simulink model "MPO_braking_system"  (R2021b)
settings: Solver=VariableStepAuto  StartTime=0.0  StopTime=10  FixedStep=0.0001  MaxStep=0.01  RelTol=1e-3  EnableMultiTasking=on
PreLoadFcn:
  | sdl_braking_caliper_disk_brake_input
InitFcn:
  | f10 = 5; f11 = f10; f12 = f10;
  | f20 = 5; f21 = f20; f22 = f20;
undefined symbols (not defined in the file or in its folder): fcdb, tpc
libraries: fl_lib x154, nesl_utility x45, SimscapeFluids_lib x6, sdl_lib x4
(part 1 of 3)
CloseFcn:
  | try,close(h_sdl_braking_caliper_disk_brake),end
  | clear h_sdl_braking_caliper_disk_brake
  | 
  | clear fcdb simT tpc tout
  | clear simlog_sdl_braking_caliper_disk_brake
settings Model: PacingRate=0.100000  Creator=samira  LastModifiedBy=109100
settings SolverCC: AlgebraicLoopSolver=TrustRegion  SolverResetMethod=Robust
settings DataIOCC: LimitDataPoints=on  SaveFormat=Array  ReturnWorkspaceOutputs=off
settings OptimizationCC: LifeSpan=inf
settings DebuggingCC: SolverPrmCheckMsg=warning  SFUnexpectedBacktrackingDiag=warning  SFNoUnconditionalDefaultTransitionDiag=warning  SFExecutionAtInitializationDiag=none  SFMachineParentedDataDiag=warning  ArithmeticOperatorsInVariantConditions=warning
settings HardwareCC: ProdBitPerPointer=32  ProdBitPerSizeT=32  ProdBitPerPtrDiffT=32  ProdLargestAtomicFloat=None  ProdIntDivRoundTo=Undefined  ProdEndianess=Unspecified  ProdWordSize=32  ProdHWDeviceType=32-bit Generic
settings ModelReferenceCC: PropagateSignalLabelsOutOfModel=off
settings SFSimCC: SimUseLocalCustomCode=off  CustomCodeUndefinedFunction=UseInterfaceOnly
settings RTWCC: RTWUseLocalCustomCode=off
settings CodeAppCC: StateflowObjectComments=on
settings GRTTargetCC: TargetLangStandard=C89/C90 (ANSI)
settings ConfigComp: CovMetricSettings=dw  CovSaveCumulativeToWorkspaceVar=on  CovSaveSingleToWorkspaceVar=on  CovExternalEMLEnable=off  CovSFcnEnable=off

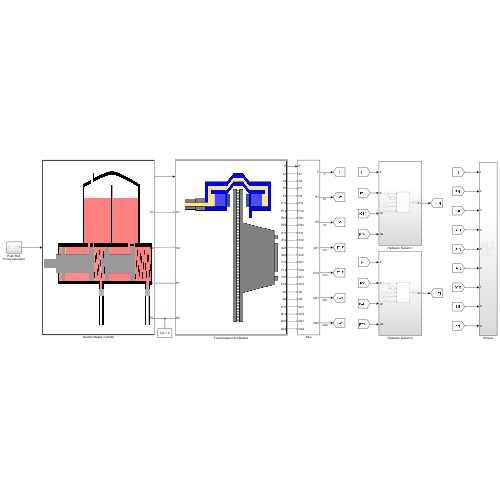
[thumbnail: Simulink's stored preview of the top-level diagram]
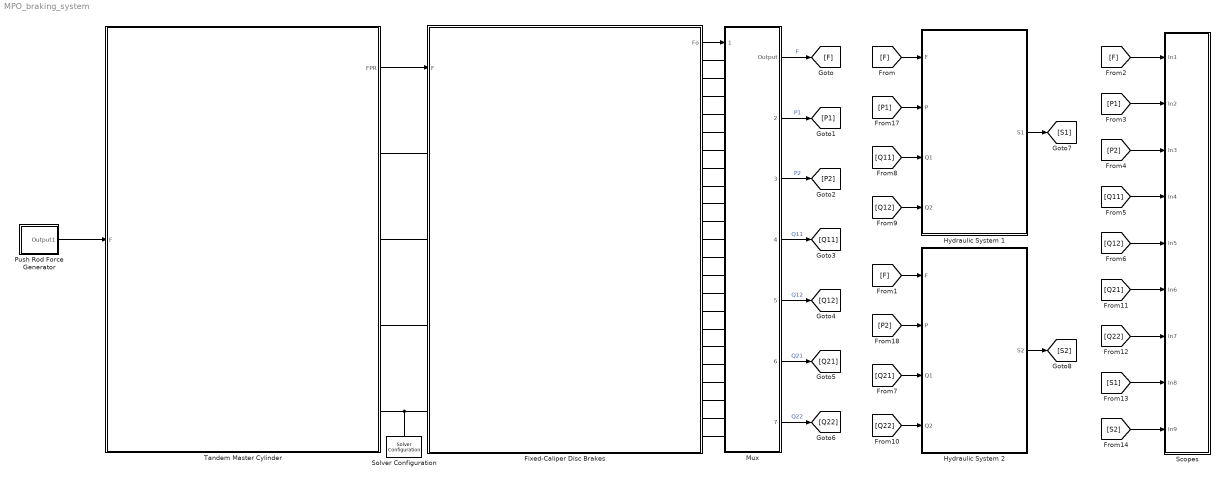
== system MPO_braking_system ==
  Fixed-Caliper Disc Brakes : Subsystem  Tag=ModelFeatures
      mask Display:
      | image('sdl_braking_caliper_disk_brake.png')
      | port_label('output',1,'F')
      | port_label('LConn',1,'X1')
      | port_label('LConn',2,'X2')
      | port_label('LConn',3,'P1')
      | port_label('LConn',4,'P2')
      | port_label('RConn',1,'X1')
      | port_label('RConn',2,'X2')
      | port_label('RConn',3,'P1')
      | port_label('RConn',4,'P2')
      | port_label('RConn',5,'P11')
      | port_label('RConn',6,'P12')
      | port_label('RConn',7,'P21')
      | port_label('RConn',8,'P22')
      | port_label('RConn',9,'X11')
      | port_label('RConn',10,'X12')
      | port_label('RConn',11,'X21')
      | port_label('RConn',12,'X22')
      | port_label('RConn',13,'F11')
      | port_label('RConn',14,'F12')
      | port_label('RConn',15,'F21')
      | port_label('RConn',16,'F22')
      | port_label('RConn',17,'Q1')
      | port_label('RConn',18,'Q2')
      | port_label('RConn',19,'Q11')
      | port_label('RConn',20,'Q12')
      | port_label('RConn',21,'Q21')
      | port_label('RConn',22,'Q22')
  Hydraulic System 1 : Subsystem
  Hydraulic System 2 : Subsystem
  Mux : Subsystem  Tag=ModelFeatures
      mask Display:
      | port_label('input',1,'F')
      | port_label('LConn',1,'S1')
      | port_label('LConn',2,'S2')
      | port_label('LConn',3,'P1')
      | port_label('LConn',4,'P2')
      | port_label('LConn',5,'P11')
      | port_label('LConn',6,'P12')
      | port_label('LConn',7,'P21')
      | port_label('LConn',8,'P22')
      | port_label('LConn',9,'S11')
      | port_label('LConn',10,'S12')
      | port_label('LConn',11,'S11')
      | port_label('LConn',12,'S12')
      | port_label('LConn',13,'Q11')
      | port_label('LConn',14,'Q12')
      | port_label('LConn',15,'Q11')
      | port_label('LConn',16,'Q12')
      | port_label('LConn',17,'Q1')
      | port_label('LConn',18,'Q2')
      | port_label('LConn',19,'Q11')
      | port_label('LConn',20,'Q12')
      | port_label('LConn',21,'Q21')
      | port_label('LConn',22,'Q22')
      | port_label('output',1,'F')
      | port_label('output',2,'P1')
      | port_label('output',3,'P2')
      | port_label('output',4,'Q11')
      | port_label('output',5,'Q12')
      | port_label('output',6,'Q21')
      | port_label('output',7,'Q22')
  Push Rod Force Generator : Subsystem
  Scopes : Subsystem
  Solver Configuration : nesl_utility/Solver Configuration  Tag=ModelFeatures  PhysicalDomain=network_engine_domain  SubClassName=solver  LeftPortType=input  RightPortType=generic  Tones=[]  Harmonics=[]  SimulateNoise=off  Profile=off  UseLocalSampling=off  EnableSwitchedLinearOptims=on  FrequencyDomain=off  UseCCode=off  RelTol=0.001  AbsTol=1e-06  MinStep=1e-09  ToWorkspace=off  RevertToSquareIcSolve=off  NumHomotopyIterations=100  PhasorMode=off  PhasorModeNumHarmonics=1  DoDC=on  ResidualTolerance=1e-09  UseLocalSolver=off  LocalSolverChoice=NE_BACKWARD_EULER_ADVANCER  LocalSolverSampleTime=0.001  DoFixedCost=off  MaxNonlinIter=3  MaxModeIter=2  ComputeImpulses=off  ImpulseIterations=2  LinearAlgebra=auto  EquationFormulation=NE_TIME_EF  DelaysMemoryBudget=1024  AutomaticFiltering=on  FilteringTimeConstant=0.001  PartitionStorageMethod=AS_NEEDED  PartitionMemoryBudget=1024  PartitionMethod=FAST
      settings: SourceProductBaseCode=PW,SS
  Tandem Master Cylinder : Subsystem
      mask Display:
      | image('sdl_braking_tandem_primary_cylinder.png');
      | %port_label('RConn',1,'F')
      | port_label('RConn',1,'X1')
      | port_label('RConn',2,'X2')
      | port_label('RConn',3,'P1')
      | port_label('RConn',4,'P2')
  wires:
  Push Rod Force Generator/1(Output1) -> Tandem Master Cylinder/1(F)
  Mux/4(Output3) -> [Q11]  "Q11"
  Tandem Master Cylinder/1(FPR) -> Fixed-Caliper Disc Brakes/1(F)
  Fixed-Caliper Disc Brakes/1(Fo) -> Mux/1(input01)
  Mux/1(Output) -> [F]  "F"
  Mux/5(Output4) -> [Q12]  "Q12"
  Mux/7(Output6) -> [Q22]  "Q22"
  Mux/6(Output5) -> [Q21]  "Q21"
  [F] -> Hydraulic System 1/1(F)
  [Q12] -> Hydraulic System 1/4(Q2)
  [Q21] -> Hydraulic System 2/3(Q1)
  [F] -> Hydraulic System 2/1(F)
  [Q22] -> Hydraulic System 2/4(Q2)
  Mux/2(Output1) -> [P1]  "P1"
  Mux/3(Output2) -> [P2]  "P2"
  [P1] -> Hydraulic System 1/2(P)
  [Q11] -> Hydraulic System 1/3(Q1)
  [P2] -> Hydraulic System 2/2(P)
  Hydraulic System 1/1(S1) -> [S1]
  Hydraulic System 2/1(S2) -> [S2]
  [F] -> Scopes/1(In1)
  [P1] -> Scopes/2(In2)
  [P2] -> Scopes/3(In3)
  [Q11] -> Scopes/4(In4)
  [Q12] -> Scopes/5(In5)
  [Q21] -> Scopes/6(In6)
  [Q22] -> Scopes/7(In7)
  [S1] -> Scopes/8(In8)
  [S2] -> Scopes/9(In9)
  connections:
  Fixed-Caliper Disc Brakes/LConn4 -- Tandem Master Cylinder/RConn4 -- Solver Configuration/RConn1
  Mux/LConn3 -- Fixed-Caliper Disc Brakes/RConn3
  Fixed-Caliper Disc Brakes/RConn19 -- Mux/LConn19
  Fixed-Caliper Disc Brakes/RConn20 -- Mux/LConn20
  Fixed-Caliper Disc Brakes/RConn21 -- Mux/LConn21
  Fixed-Caliper Disc Brakes/LConn3 -- Tandem Master Cylinder/RConn3
  Tandem Master Cylinder/RConn1 -- Fixed-Caliper Disc Brakes/LConn1
  Mux/LConn4 -- Fixed-Caliper Disc Brakes/RConn4
  Tandem Master Cylinder/RConn2 -- Fixed-Caliper Disc Brakes/LConn2
  Fixed-Caliper Disc Brakes/RConn18 -- Mux/LConn18
  Fixed-Caliper Disc Brakes/RConn17 -- Mux/LConn17
  Fixed-Caliper Disc Brakes/RConn16 -- Mux/LConn16
  Fixed-Caliper Disc Brakes/RConn15 -- Mux/LConn15
  Fixed-Caliper Disc Brakes/RConn14 -- Mux/LConn14
  Fixed-Caliper Disc Brakes/RConn13 -- Mux/LConn13
  Mux/LConn12 -- Fixed-Caliper Disc Brakes/RConn12
  Fixed-Caliper Disc Brakes/RConn11 -- Mux/LConn11
  Fixed-Caliper Disc Brakes/RConn10 -- Mux/LConn10
  Fixed-Caliper Disc Brakes/RConn9 -- Mux/LConn9
  Fixed-Caliper Disc Brakes/RConn1 -- Mux/LConn1
  Fixed-Caliper Disc Brakes/RConn2 -- Mux/LConn2
  Fixed-Caliper Disc Brakes/RConn5 -- Mux/LConn5
  Fixed-Caliper Disc Brakes/RConn6 -- Mux/LConn6
  Fixed-Caliper Disc Brakes/RConn7 -- Mux/LConn7
  Fixed-Caliper Disc Brakes/RConn8 -- Mux/LConn8
  Fixed-Caliper Disc Brakes/RConn22 -- Mux/LConn22

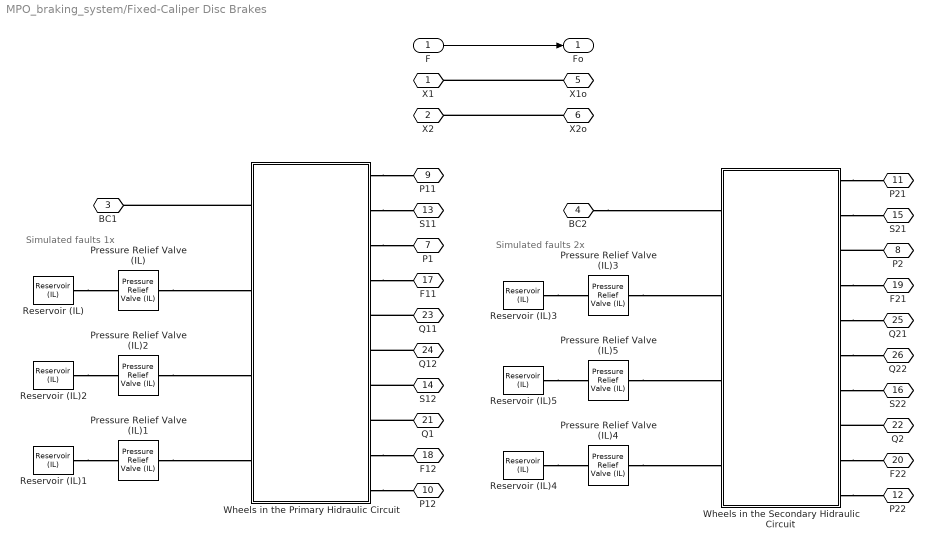
== system MPO_braking_system/Fixed-Caliper Disc Brakes ==
  note: Simulated faults 1x
  note: Simulated faults 2x
  F : Inport
  Pressure Relief Valve (IL) : SimscapeFluids_lib/Isothermal Liquid/Valves & Orifices/Pressure Control Valves/Pressure Relief Valve (IL)  set_pressure_spec=foundation.enum.constant_controlled.constant  pressure_spec=fluids.isothermal_liquid.valves_orifices.enum.pressure_control_spec.dp  p_set_gauge=0.1 MPa  p_set_differential=f10 MPa  p_range=0.1 MPa  opening_spec=fluids.isothermal_liquid.valves_orifices.enum.opening_spec.linear  area_max=1e-4 m^2  area_leak=1e-10 m^2  p_diff_TLU=[0.2 : 0.2 : 1.2] MPa  valve_area_TLU=[1e-10, 2e-06, 4e-06, 6e-06, 8e-06, 1e-05] m^2  area=inf m^2  Cd=0.64  Re_c=150  pressure_recovery=simscape.enum.onoff.off  smoothing_factor=0.01  opening_dynamics=simscape.enum.onoff.off  tau=0.1 s  enable_faults=simscape.enum.onoff.off  fault_type=fluids.enum.FaultOpening.Closed  fault_trigger=foundation.enum.faultSpec.Temporal  fault_time=5 s
      settings: SourceProductBaseCode=SH  InternalSimscapePortConfiguration="{\"Bottom\":[],\"Left\":[{\"id\":\"A\",\"label\":\"A\",\"type\":\"foundation.isothermal_liquid.isothermal_liquid\"}],\"Right\":[{\"id\":\"B\",\"label\":\"B\",\"type\":\"foundation.isothermal_liquid.isothermal_liquid\"}],\"Top\":[]}"
  Pressure Relief Valve (IL)1 : SimscapeFluids_lib/Isothermal Liquid/Valves & Orifices/Pressure Control Valves/Pressure Relief Valve (IL)  set_pressure_spec=foundation.enum.constant_controlled.constant  pressure_spec=fluids.isothermal_liquid.valves_orifices.enum.pressure_control_spec.dp  p_set_gauge=0.1 MPa  p_set_differential=f12 MPa  p_range=0.1 MPa  opening_spec=fluids.isothermal_liquid.valves_orifices.enum.opening_spec.linear  area_max=1e-4 m^2  area_leak=1e-10 m^2  p_diff_TLU=[0.2 : 0.2 : 1.2] MPa  valve_area_TLU=[1e-10, 2e-06, 4e-06, 6e-06, 8e-06, 1e-05] m^2  area=inf m^2  Cd=0.64  Re_c=150  pressure_recovery=simscape.enum.onoff.off  smoothing_factor=0.01  opening_dynamics=simscape.enum.onoff.off  tau=0.1 s  enable_faults=simscape.enum.onoff.off  fault_type=fluids.enum.FaultOpening.Closed  fault_trigger=foundation.enum.faultSpec.Temporal  fault_time=5 s
      settings: SourceProductBaseCode=SH  InternalSimscapePortConfiguration="{\"Bottom\":[],\"Left\":[{\"id\":\"A\",\"label\":\"A\",\"type\":\"foundation.isothermal_liquid.isothermal_liquid\"}],\"Right\":[{\"id\":\"B\",\"label\":\"B\",\"type\":\"foundation.isothermal_liquid.isothermal_liquid\"}],\"Top\":[]}"
  Pressure Relief Valve (IL)2 : SimscapeFluids_lib/Isothermal Liquid/Valves & Orifices/Pressure Control Valves/Pressure Relief Valve (IL)  set_pressure_spec=foundation.enum.constant_controlled.constant  pressure_spec=fluids.isothermal_liquid.valves_orifices.enum.pressure_control_spec.dp  p_set_gauge=0.1 MPa  p_set_differential=f11 MPa  p_range=0.1 MPa  opening_spec=fluids.isothermal_liquid.valves_orifices.enum.opening_spec.linear  area_max=1e-4 m^2  area_leak=1e-10 m^2  p_diff_TLU=[0.2 : 0.2 : 1.2] MPa  valve_area_TLU=[1e-10, 2e-06, 4e-06, 6e-06, 8e-06, 1e-05] m^2  area=inf m^2  Cd=0.64  Re_c=150  pressure_recovery=simscape.enum.onoff.off  smoothing_factor=0.01  opening_dynamics=simscape.enum.onoff.off  tau=0.1 s  enable_faults=simscape.enum.onoff.off  fault_type=fluids.enum.FaultOpening.Closed  fault_trigger=foundation.enum.faultSpec.Temporal  fault_time=5 s
      settings: SourceProductBaseCode=SH  InternalSimscapePortConfiguration="{\"Bottom\":[],\"Left\":[{\"id\":\"A\",\"label\":\"A\",\"type\":\"foundation.isothermal_liquid.isothermal_liquid\"}],\"Right\":[{\"id\":\"B\",\"label\":\"B\",\"type\":\"foundation.isothermal_liquid.isothermal_liquid\"}],\"Top\":[]}"
  Pressure Relief Valve (IL)3 : SimscapeFluids_lib/Isothermal Liquid/Valves & Orifices/Pressure Control Valves/Pressure Relief Valve (IL)  set_pressure_spec=foundation.enum.constant_controlled.constant  pressure_spec=fluids.isothermal_liquid.valves_orifices.enum.pressure_control_spec.dp  p_set_gauge=0.1 MPa  p_set_differential=f20 MPa  p_range=0.1 MPa  opening_spec=fluids.isothermal_liquid.valves_orifices.enum.opening_spec.linear  area_max=1e-4 m^2  area_leak=1e-10 m^2  p_diff_TLU=[0.2 : 0.2 : 1.2] MPa  valve_area_TLU=[1e-10, 2e-06, 4e-06, 6e-06, 8e-06, 1e-05] m^2  area=inf m^2  Cd=0.64  Re_c=150  pressure_recovery=simscape.enum.onoff.off  smoothing_factor=0.01  opening_dynamics=simscape.enum.onoff.off  tau=0.1 s  enable_faults=simscape.enum.onoff.off  fault_type=fluids.enum.FaultOpening.Closed  fault_trigger=foundation.enum.faultSpec.Temporal  fault_time=5 s
      settings: SourceProductBaseCode=SH  InternalSimscapePortConfiguration="{\"Bottom\":[],\"Left\":[{\"id\":\"A\",\"label\":\"A\",\"type\":\"foundation.isothermal_liquid.isothermal_liquid\"}],\"Right\":[{\"id\":\"B\",\"label\":\"B\",\"type\":\"foundation.isothermal_liquid.isothermal_liquid\"}],\"Top\":[]}"
  Pressure Relief Valve (IL)4 : SimscapeFluids_lib/Isothermal Liquid/Valves & Orifices/Pressure Control Valves/Pressure Relief Valve (IL)  set_pressure_spec=foundation.enum.constant_controlled.constant  pressure_spec=fluids.isothermal_liquid.valves_orifices.enum.pressure_control_spec.dp  p_set_gauge=0.1 MPa  p_set_differential=f22 MPa  p_range=0.1 MPa  opening_spec=fluids.isothermal_liquid.valves_orifices.enum.opening_spec.linear  area_max=1e-4 m^2  area_leak=1e-10 m^2  p_diff_TLU=[0.2 : 0.2 : 1.2] MPa  valve_area_TLU=[1e-10, 2e-06, 4e-06, 6e-06, 8e-06, 1e-05] m^2  area=inf m^2  Cd=0.64  Re_c=150  pressure_recovery=simscape.enum.onoff.off  smoothing_factor=0.01  opening_dynamics=simscape.enum.onoff.off  tau=0.1 s  enable_faults=simscape.enum.onoff.off  fault_type=fluids.enum.FaultOpening.Closed  fault_trigger=foundation.enum.faultSpec.Temporal  fault_time=5 s
      settings: SourceProductBaseCode=SH  InternalSimscapePortConfiguration="{\"Bottom\":[],\"Left\":[{\"id\":\"A\",\"label\":\"A\",\"type\":\"foundation.isothermal_liquid.isothermal_liquid\"}],\"Right\":[{\"id\":\"B\",\"label\":\"B\",\"type\":\"foundation.isothermal_liquid.isothermal_liquid\"}],\"Top\":[]}"
  Pressure Relief Valve (IL)5 : SimscapeFluids_lib/Isothermal Liquid/Valves & Orifices/Pressure Control Valves/Pressure Relief Valve (IL)  set_pressure_spec=foundation.enum.constant_controlled.constant  pressure_spec=fluids.isothermal_liquid.valves_orifices.enum.pressure_control_spec.dp  p_set_gauge=0.1 MPa  p_set_differential=f21 MPa  p_range=0.1 MPa  opening_spec=fluids.isothermal_liquid.valves_orifices.enum.opening_spec.linear  area_max=1e-4 m^2  area_leak=1e-10 m^2  p_diff_TLU=[0.2 : 0.2 : 1.2] MPa  valve_area_TLU=[1e-10, 2e-06, 4e-06, 6e-06, 8e-06, 1e-05] m^2  area=inf m^2  Cd=0.64  Re_c=150  pressure_recovery=simscape.enum.onoff.off  smoothing_factor=0.01  opening_dynamics=simscape.enum.onoff.off  tau=0.1 s  enable_faults=simscape.enum.onoff.off  fault_type=fluids.enum.FaultOpening.Closed  fault_trigger=foundation.enum.faultSpec.Temporal  fault_time=5 s
      settings: SourceProductBaseCode=SH  InternalSimscapePortConfiguration="{\"Bottom\":[],\"Left\":[{\"id\":\"A\",\"label\":\"A\",\"type\":\"foundation.isothermal_liquid.isothermal_liquid\"}],\"Right\":[{\"id\":\"B\",\"label\":\"B\",\"type\":\"foundation.isothermal_liquid.isothermal_liquid\"}],\"Top\":[]}"
  Reservoir (IL){,1..5} (6 alike) : fl_lib/Isothermal Liquid/Elements/Reservoir (IL)  reservoir_type=foundation.enum.constant_controlled.constant  pressure_spec=foundation.enum.pressure_spec.atmospheric  reservoir_pressure=0.101325 MPa
      settings: SourceProductBaseCode=SS
  Wheels in the Primary Hidraulic Circuit : Subsystem
  Wheels in the Secondary Hidraulic Circuit : Subsystem
  X1 : PMIOPort  Side=Left
  X2 : PMIOPort  Port=2  Side=Left
  BC1 : PMIOPort  Port=3  Side=Left
  BC2 : PMIOPort  Port=4  Side=Left
  X1o : PMIOPort  Port=5  Side=Right
  X2o : PMIOPort  Port=6  Side=Right
  P1 : PMIOPort  Port=7  Side=Right
  P2 : PMIOPort  Port=8  Side=Right
  P11 : PMIOPort  Port=9  Side=Right
  P12 : PMIOPort  Port=10  Side=Right
  P21 : PMIOPort  Port=11  Side=Right
  P22 : PMIOPort  Port=12  Side=Right
  S11 : PMIOPort  Port=13  Side=Right
  S12 : PMIOPort  Port=14  Side=Right
  S21 : PMIOPort  Port=15  Side=Right
  S22 : PMIOPort  Port=16  Side=Right
  F11 : PMIOPort  Port=17  Side=Right
  F12 : PMIOPort  Port=18  Side=Right
  F21 : PMIOPort  Port=19  Side=Right
  F22 : PMIOPort  Port=20  Side=Right
  Q1 : PMIOPort  Port=21  Side=Right
  Q2 : PMIOPort  Port=22  Side=Right
  Q11 : PMIOPort  Port=23  Side=Right
  Q12 : PMIOPort  Port=24  Side=Right
  Q21 : PMIOPort  Port=25  Side=Right
  Q22 : PMIOPort  Port=26  Side=Right
  Fo : Outport
  wires:
  F/1 -> Fo/1
  connections:
  X1o/RConn1 -- X1/RConn1
  X2o/RConn1 -- X2/RConn1
  Reservoir (IL)/LConn1 -- Pressure Relief Valve (IL)/RConn1
  Reservoir (IL)2/LConn1 -- Pressure Relief Valve (IL)2/RConn1
  Reservoir (IL)1/LConn1 -- Pressure Relief Valve (IL)1/RConn1
  Reservoir (IL)5/LConn1 -- Pressure Relief Valve (IL)5/RConn1
  Reservoir (IL)3/LConn1 -- Pressure Relief Valve (IL)3/RConn1
  Reservoir (IL)4/LConn1 -- Pressure Relief Valve (IL)4/RConn1
  Wheels in the Primary Hidraulic Circuit/RConn1 -- P11/RConn1
  Wheels in the Primary Hidraulic Circuit/RConn2 -- S11/RConn1
  Wheels in the Primary Hidraulic Circuit/RConn3 -- P1/RConn1
  Wheels in the Primary Hidraulic Circuit/RConn4 -- F11/RConn1
  Q11/RConn1 -- Wheels in the Primary Hidraulic Circuit/RConn5
  Wheels in the Primary Hidraulic Circuit/LConn1 -- BC1/RConn1
  Q12/RConn1 -- Wheels in the Primary Hidraulic Circuit/RConn6
  S12/RConn1 -- Wheels in the Primary Hidraulic Circuit/RConn7
  Q1/RConn1 -- Wheels in the Primary Hidraulic Circuit/RConn8
  Wheels in the Primary Hidraulic Circuit/RConn9 -- F12/RConn1
  Wheels in the Primary Hidraulic Circuit/RConn10 -- P12/RConn1
  Pressure Relief Valve (IL)/LConn1 -- Wheels in the Primary Hidraulic Circuit/LConn2
  Pressure Relief Valve (IL)2/LConn1 -- Wheels in the Primary Hidraulic Circuit/LConn3
  Pressure Relief Valve (IL)1/LConn1 -- Wheels in the Primary Hidraulic Circuit/LConn4
  Wheels in the Secondary Hidraulic Circuit/RConn1 -- P21/RConn1
  Wheels in the Secondary Hidraulic Circuit/RConn2 -- S21/RConn1
  P2/RConn1 -- Wheels in the Secondary Hidraulic Circuit/RConn3
  Wheels in the Secondary Hidraulic Circuit/RConn4 -- F21/RConn1
  Wheels in the Secondary Hidraulic Circuit/RConn5 -- Q21/RConn1
  BC2/RConn1 -- Wheels in the Secondary Hidraulic Circuit/LConn1
  Wheels in the Secondary Hidraulic Circuit/RConn6 -- Q22/RConn1
  Wheels in the Secondary Hidraulic Circuit/RConn7 -- S22/RConn1
  Q2/RConn1 -- Wheels in the Secondary Hidraulic Circuit/RConn8
  Wheels in the Secondary Hidraulic Circuit/RConn9 -- F22/RConn1
  Wheels in the Secondary Hidraulic Circuit/RConn10 -- P22/RConn1
  Pressure Relief Valve (IL)3/LConn1 -- Wheels in the Secondary Hidraulic Circuit/LConn2
  Pressure Relief Valve (IL)5/LConn1 -- Wheels in the Secondary Hidraulic Circuit/LConn3
  Pressure Relief Valve (IL)4/LConn1 -- Wheels in the Secondary Hidraulic Circuit/LConn4

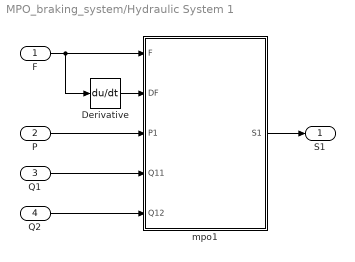
== system MPO_braking_system/Hydraulic System 1 ==
  F : Inport
  P : Inport  Port=2
  Q1 : Inport  Port=3
  Q2 : Inport  Port=4
  Derivative : Derivative
  mpo1 : Stateflow chart  TreatAsAtomicUnit=on
  S1 : Outport
  wires:
  Derivative/1 -> mpo1/2(DF)
  Q2/1 -> mpo1/5(Q12)
  F/1 -> mpo1/1(F), Derivative/1
  Q1/1 -> mpo1/4(Q11)
  P/1 -> mpo1/3(P1)
  mpo1/1(S1) -> S1/1

== system MPO_braking_system/Hydraulic System 2 ==
  F : Inport
  P : Inport  Port=2
  Q1 : Inport  Port=3
  Q2 : Inport  Port=4
  Derivative : Derivative
  mpo2 : Stateflow chart  TreatAsAtomicUnit=on
  S2 : Outport
  wires:
  Derivative/1 -> mpo2/2(DF)
  Q2/1 -> mpo2/5(Q12)
  F/1 -> mpo2/1(F), Derivative/1
  Q1/1 -> mpo2/4(Q11)
  P/1 -> mpo2/3(P1)
  mpo2/1(S2) -> S2/1

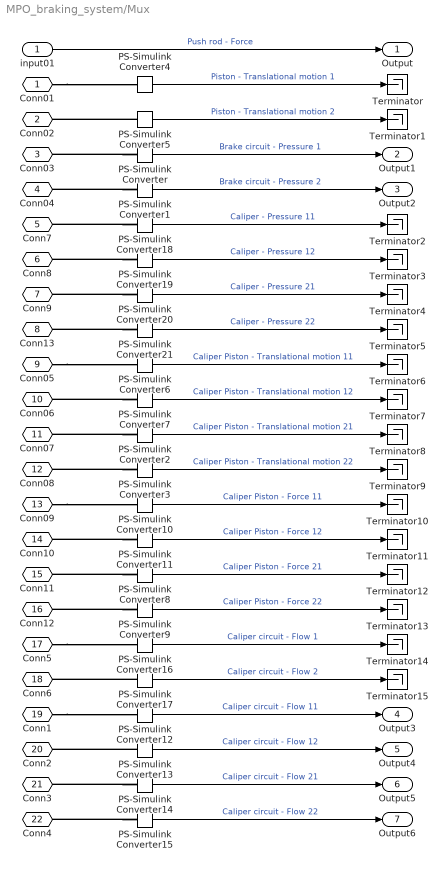
== system MPO_braking_system/Mux ==
  input01 : Inport
  PS-Simulink Converter{,1,18..21} (6 alike) : nesl_utility/PS-Simulink Converter  PhysicalDomain=network_engine_domain  SubClassName=ps_output  LeftPortType=input  RightPortType=output  PseudoPeriodic=off  Frequencies=[]  Unit=Pa  AffineConversion=off
      settings: SourceProductBaseCode=PW,SS
  PS-Simulink Converter{8..11} (4 alike) : nesl_utility/PS-Simulink Converter  PhysicalDomain=network_engine_domain  SubClassName=ps_output  LeftPortType=input  RightPortType=output  PseudoPeriodic=off  Frequencies=[]  Unit=N  AffineConversion=off
      settings: SourceProductBaseCode=PW,SS
  PS-Simulink Converter{12..17} (6 alike) : nesl_utility/PS-Simulink Converter  PhysicalDomain=network_engine_domain  SubClassName=ps_output  LeftPortType=input  RightPortType=output  PseudoPeriodic=off  Frequencies=[]  Unit=m^3/s  AffineConversion=off
      settings: SourceProductBaseCode=PW,SS
  PS-Simulink Converter{2..7} (6 alike) : nesl_utility/PS-Simulink Converter  PhysicalDomain=network_engine_domain  SubClassName=ps_output  LeftPortType=input  RightPortType=output  PseudoPeriodic=off  Frequencies=[]  Unit=m  AffineConversion=off
      settings: SourceProductBaseCode=PW,SS
  Terminator{,1..15} (16 alike) : Terminator
  Conn01 : PMIOPort  Side=Left
  Conn02 : PMIOPort  Port=2  Side=Left
  Conn03 : PMIOPort  Port=3  Side=Left
  Conn04 : PMIOPort  Port=4  Side=Left
  Conn7 : PMIOPort  Port=5  Side=Left
  Conn8 : PMIOPort  Port=6  Side=Left
  Conn9 : PMIOPort  Port=7  Side=Left
  Conn13 : PMIOPort  Port=8  Side=Left
  Conn05 : PMIOPort  Port=9  Side=Left
  Conn06 : PMIOPort  Port=10  Side=Left
  Conn07 : PMIOPort  Port=11  Side=Left
  Conn08 : PMIOPort  Port=12  Side=Left
  Conn09 : PMIOPort  Port=13  Side=Left
  Conn10 : PMIOPort  Port=14  Side=Left
  Conn11 : PMIOPort  Port=15  Side=Left
  Conn12 : PMIOPort  Port=16  Side=Left
  Conn5 : PMIOPort  Port=17  Side=Left
  Conn6 : PMIOPort  Port=18  Side=Left
  Conn1 : PMIOPort  Port=19  Side=Left
  Conn2 : PMIOPort  Port=20  Side=Left
  Conn3 : PMIOPort  Port=21  Side=Left
  Conn4 : PMIOPort  Port=22  Side=Left
  Output : Outport
  Output1 : Outport  Port=2
  Output2 : Outport  Port=3
  Output3 : Outport  Port=4
  Output4 : Outport  Port=5
  Output5 : Outport  Port=6
  Output6 : Outport  Port=7
  wires:
  PS-Simulink Converter/1 -> Output1/1  "Brake circuit - Pressure 1"
  PS-Simulink Converter4/1 -> Terminator/1  "Piston - Translational motion 1"
  input01/1 -> Output/1  "Push rod - Force"
  PS-Simulink Converter10/1 -> Terminator10/1  "Caliper Piston - Force 11"
  PS-Simulink Converter1/1 -> Output2/1  "Brake circuit - Pressure 2"
  PS-Simulink Converter11/1 -> Terminator11/1  "Caliper Piston - Force 12"
  PS-Simulink Converter8/1 -> Terminator12/1  "Caliper Piston - Force 21"
  PS-Simulink Converter9/1 -> Terminator13/1  "Caliper Piston - Force 22"
  PS-Simulink Converter6/1 -> Terminator6/1  "Caliper Piston - Translational motion 11"
  PS-Simulink Converter7/1 -> Terminator7/1  "Caliper Piston - Translational motion 12"
  PS-Simulink Converter2/1 -> Terminator8/1  "Caliper Piston - Translational motion 21"
  PS-Simulink Converter3/1 -> Terminator9/1  "Caliper Piston - Translational motion 22"
  PS-Simulink Converter12/1 -> Output3/1  "Caliper circuit - Flow 11"
  PS-Simulink Converter13/1 -> Output4/1  "Caliper circuit - Flow 12"
  PS-Simulink Converter14/1 -> Output5/1  "Caliper circuit - Flow 21"
  PS-Simulink Converter15/1 -> Output6/1  "Caliper circuit - Flow 22"
  PS-Simulink Converter16/1 -> Terminator14/1  "Caliper circuit - Flow 1"
  PS-Simulink Converter17/1 -> Terminator15/1  "Caliper circuit - Flow 2"
  PS-Simulink Converter19/1 -> Terminator3/1  "Caliper - Pressure 12"
  PS-Simulink Converter18/1 -> Terminator2/1  "Caliper - Pressure 11"
  PS-Simulink Converter21/1 -> Terminator5/1  "Caliper - Pressure 22"
  PS-Simulink Converter20/1 -> Terminator4/1  "Caliper - Pressure 21"
  PS-Simulink Converter5/1 -> Terminator1/1  "Piston - Translational motion 2"
  connections:
  PS-Simulink Converter/LConn1 -- Conn03/RConn1
  PS-Simulink Converter1/LConn1 -- Conn04/RConn1
  PS-Simulink Converter5/LConn1 -- Conn02/RConn1
  Conn01/RConn1 -- PS-Simulink Converter4/LConn1
  PS-Simulink Converter7/LConn1 -- Conn06/RConn1
  PS-Simulink Converter2/LConn1 -- Conn07/RConn1
  Conn05/RConn1 -- PS-Simulink Converter6/LConn1
  PS-Simulink Converter3/LConn1 -- Conn08/RConn1
  PS-Simulink Converter11/LConn1 -- Conn10/RConn1
  PS-Simulink Converter8/LConn1 -- Conn11/RConn1
  PS-Simulink Converter9/LConn1 -- Conn12/RConn1
  Conn09/RConn1 -- PS-Simulink Converter10/LConn1
  PS-Simulink Converter14/LConn1 -- Conn3/RConn1
  Conn1/RConn1 -- PS-Simulink Converter12/LConn1
  PS-Simulink Converter13/LConn1 -- Conn2/RConn1
  PS-Simulink Converter15/LConn1 -- Conn4/RConn1
  PS-Simulink Converter17/LConn1 -- Conn6/RConn1
  Conn5/RConn1 -- PS-Simulink Converter16/LConn1
  PS-Simulink Converter19/LConn1 -- Conn8/RConn1
  PS-Simulink Converter18/LConn1 -- Conn7/RConn1
  PS-Simulink Converter21/LConn1 -- Conn13/RConn1
  PS-Simulink Converter20/LConn1 -- Conn9/RConn1

== system MPO_braking_system/Push Rod Force Generator ==
  Clock : Clock
  Constant : Constant  Value=10e3
  Force Generation : MATLAB Function  TreatAsAtomicUnit=on
  Saturation : Saturate  UpperLimit=tpc.pushRodF(3)  LowerLimit=0
  Stop Simulation : Stop
  Output1 : Outport
  wires:
  Saturation/1 -> Output1/1
  Clock/1 -> Force Generation/1(clock)
  Force Generation/2(signal) -> Saturation/1
  Force Generation/1(stop) -> Stop Simulation/1
  Constant/1 -> Force Generation/2(rate)

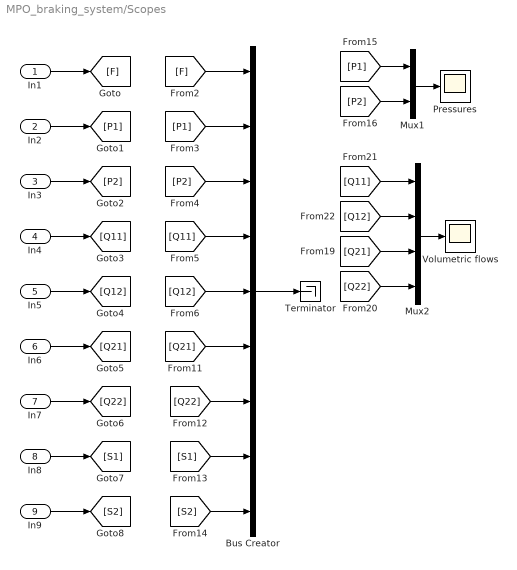
== system MPO_braking_system/Scopes ==
  In1 : Inport
  In2 : Inport  Port=2
  In3 : Inport  Port=3
  In4 : Inport  Port=4
  In5 : Inport  Port=5
  In6 : Inport  Port=6
  In7 : Inport  Port=7
  In8 : Inport  Port=8
  In9 : Inport  Port=9
  Bus Creator : BusCreator  Inputs=9
  Mux1 : Mux  Inputs=2
  Mux2 : Mux
  Pressures : Scope
  Terminator : Terminator
  Volumetric flows : Scope
  wires:
  [Q12] -> Mux2/2
  Bus Creator/1 -> Terminator/1
  In3/1 -> [P2]
  [Q21] -> Mux2/3
  Mux2/1 -> Volumetric flows/1
  In6/1 -> [Q21]
  [Q22] -> Mux2/4
  [P2] -> Mux1/2
  [Q11] -> Mux2/1
  [P1] -> Mux1/1
  In8/1 -> [S1]
  Mux1/1 -> Pressures/1
  In2/1 -> [P1]
  In4/1 -> [Q11]
  In1/1 -> [F]
  In5/1 -> [Q12]
  [S1] -> Bus Creator/8
  [Q21] -> Bus Creator/6
  [Q11] -> Bus Creator/4
  [Q12] -> Bus Creator/5
  [F] -> Bus Creator/1
  [P2] -> Bus Creator/3
  [Q22] -> Bus Creator/7
  [P1] -> Bus Creator/2
  [S2] -> Bus Creator/9
  In7/1 -> [Q22]
  In9/1 -> [S2]

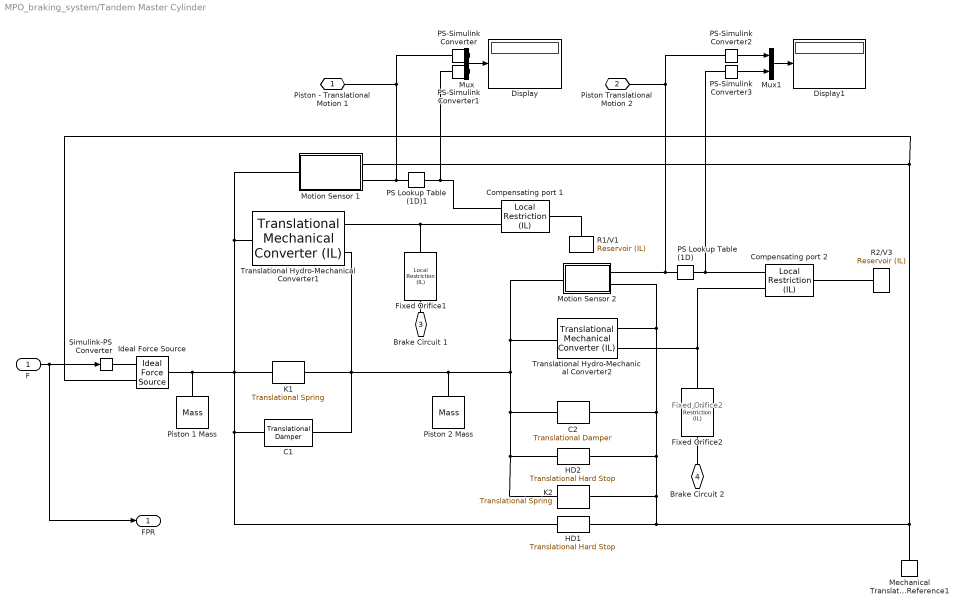
== system MPO_braking_system/Tandem Master Cylinder ==
  note: Fixed Orifice2
  F : Inport
  C1 : fl_lib/Mechanical/Translational Elements/Translational Damper  D=tpc.c1 N/(m/s)  v_specify=off  v_priority=None  v=0 m/s  v_nominal_specify=off  v_nominal_unit=m/s  v_nominal_value=1  f_specify=off  f_priority=None  f=0 N  f_nominal_specify=off  f_nominal_unit=N  f_nominal_value=1
  C2 : fl_lib/Mechanical/Translational Elements/Translational Damper  D=tpc.c2 N/(m/s)  v_specify=off  v_priority=None  v=0 m/s  v_nominal_specify=off  v_nominal_unit=m/s  v_nominal_value=1  f_specify=off  f_priority=None  f=0 N  f_nominal_specify=off  f_nominal_unit=N  f_nominal_value=1
  Compensating port 1 : fl_lib/Isothermal Liquid/Elements/Local Restriction (IL)  restriction_type=foundation.enum.restriction_type.variable  restriction_area=1e-3 m^2  min_area=1e-15 m^2  max_area="tpc.a1Ori  m^2"  area=inf m^2  Cd=0.7  Re_c=150  pressure_recovery=simscape.enum.onoff.off
      settings: SourceProductBaseCode=SS  InternalSimscapePortConfiguration="{\"Bottom\":[],\"Left\":[{\"id\":\"A\",\"label\":\"A\",\"type\":\"foundation.isothermal_liquid.isothermal_liquid\"},{\"id\":\"AR\",\"label\":\"AR\",\"type\":\"input\"}],\"Right\":[{\"id\":\"B\",\"label\":\"B\",\"type\":\"foundation.isothermal_liquid.isothermal_liquid\"}],\"Top\":[]}"
  Compensating port 2 : fl_lib/Isothermal Liquid/Elements/Local Restriction (IL)  restriction_type=foundation.enum.restriction_type.variable  restriction_area=1e-3 m^2  min_area=1e-15 m^2  max_area="tpc.a1Ori  m^2"  area=inf m^2  Cd=0.7  Re_c=150  pressure_recovery=simscape.enum.onoff.off
      settings: SourceProductBaseCode=SS  InternalSimscapePortConfiguration="{\"Bottom\":[],\"Left\":[{\"id\":\"A\",\"label\":\"A\",\"type\":\"foundation.isothermal_liquid.isothermal_liquid\"},{\"id\":\"AR\",\"label\":\"AR\",\"type\":\"input\"}],\"Right\":[{\"id\":\"B\",\"label\":\"B\",\"type\":\"foundation.isothermal_liquid.isothermal_liquid\"}],\"Top\":[]}"
  Display : Display
  Display1 : Display
  Fixed Orifice1 : fl_lib/Isothermal Liquid/Elements/Local Restriction (IL)  restriction_type=foundation.enum.restriction_type.fixed  restriction_area=tpc.a2Ori m^2  min_area=1e-15 m^2  max_area="tpc.a1Ori  m^2"  area=inf m^2  Cd=0.7  Re_c=150  pressure_recovery=simscape.enum.onoff.off
      settings: SourceProductBaseCode=SS  InternalSimscapePortConfiguration="{\"Bottom\":[],\"Left\":[{\"id\":\"A\",\"label\":\"A\",\"type\":\"foundation.isothermal_liquid.isothermal_liquid\"}],\"Right\":[{\"id\":\"B\",\"label\":\"B\",\"type\":\"foundation.isothermal_liquid.isothermal_liquid\"}],\"Top\":[]}"
  Fixed Orifice2 : fl_lib/Isothermal Liquid/Elements/Local Restriction (IL)  restriction_type=foundation.enum.restriction_type.fixed  restriction_area=tpc.a2Ori m^2  min_area=1e-15 m^2  max_area="tpc.a1Ori  m^2"  area=inf m^2  Cd=0.7  Re_c=150  pressure_recovery=simscape.enum.onoff.off
      settings: SourceProductBaseCode=SS  InternalSimscapePortConfiguration="{\"Bottom\":[],\"Left\":[{\"id\":\"A\",\"label\":\"A\",\"type\":\"foundation.isothermal_liquid.isothermal_liquid\"}],\"Right\":[{\"id\":\"B\",\"label\":\"B\",\"type\":\"foundation.isothermal_liquid.isothermal_liquid\"}],\"Top\":[]}"
  HD1 : fl_lib/Mechanical/Translational Elements/Translational Hard Stop  upper_bnd=tpc.x13 m  lower_bnd=0 m  stiff_up=tpc.hss N/m  stiff_low=tpc.hss N/m  D_up=tpc.hsd N/(m/s)  D_low=tpc.hsd N/(m/s)  model=simscape.enum.hardstop.smooth  transition=0.1 mm  v_specify=off  v_priority=None  v=0 m/s  v_nominal_specify=off  v_nominal_unit=m/s  v_nominal_value=1  f_specify=off  f_priority=None  f=0 N  f_nominal_specify=off  f_nominal_unit=N  f_nominal_value=1  x_specify=off  x_priority=High  x=0 m  x_nominal_specify=off  x_nominal_unit=m  x_nominal_value=1
  HD2 : fl_lib/Mechanical/Translational Elements/Translational Hard Stop  upper_bnd=tpc.x23 m  lower_bnd=0 m  stiff_up=tpc.hss N/m  stiff_low=tpc.hss N/m  D_up=tpc.hsd N/(m/s)  D_low=tpc.hsd N/(m/s)  model=simscape.enum.hardstop.smooth  transition=0.1 mm  v_specify=off  v_priority=None  v=0 m/s  v_nominal_specify=off  v_nominal_unit=m/s  v_nominal_value=1  f_specify=off  f_priority=None  f=0 N  f_nominal_specify=off  f_nominal_unit=N  f_nominal_value=1  x_specify=off  x_priority=High  x=0 m  x_nominal_specify=off  x_nominal_unit=m  x_nominal_value=1
  Ideal Force Source : fl_lib/Mechanical/Mechanical Sources/Ideal Force Source
  K1 : fl_lib/Mechanical/Translational Elements/Translational Spring  spr_rate=tpc.k1 N/m  v_specify=off  v_priority=None  v=0 m/s  v_nominal_specify=off  v_nominal_unit=m/s  v_nominal_value=1  f_specify=off  f_priority=None  f=0 N  f_nominal_specify=off  f_nominal_unit=N  f_nominal_value=1  x_specify=on  x_priority=High  x=tpc.defLL m  x_nominal_specify=off  x_nominal_unit=m  x_nominal_value=1
  K2 : fl_lib/Mechanical/Translational Elements/Translational Spring  spr_rate=tpc.k2 N/m  v_specify=off  v_priority=None  v=0 m/s  v_nominal_specify=off  v_nominal_unit=m/s  v_nominal_value=1  f_specify=off  f_priority=None  f=0 N  f_nominal_specify=off  f_nominal_unit=N  f_nominal_value=1  x_specify=on  x_priority=High  x=tpc.defLR m  x_nominal_specify=off  x_nominal_unit=m  x_nominal_value=1
  Mechanical Translational Reference1 : fl_lib/Mechanical/Translational Elements/Mechanical Translational Reference
  Motion Sensor 1 : Subsystem
  Motion Sensor 2 : Subsystem
  Mux : Mux  Inputs=2
  Mux1 : Mux  Inputs=2
  PS Lookup Table (1D) : fl_lib/Physical Signals/Lookup Tables/PS Lookup Table (1D)  x=[0 tpc.x22 tpc.x23] m  f=[tpc.a1Ori 0 0] m^2  interp_method=simscape.enum.interpolation.linear  extrap_method=simscape.enum.extrapolation.linear
      settings: SourceProductBaseCode=SS
  PS Lookup Table (1D)1 : fl_lib/Physical Signals/Lookup Tables/PS Lookup Table (1D)  x=[0 tpc.x12 tpc.x13] m  f=[tpc.a1Ori 0 0] m^2  interp_method=simscape.enum.interpolation.linear  extrap_method=simscape.enum.extrapolation.linear
      settings: SourceProductBaseCode=SS
  PS-Simulink Converter{,1..3} (4 alike) : nesl_utility/PS-Simulink Converter  PhysicalDomain=network_engine_domain  SubClassName=ps_output  LeftPortType=input  RightPortType=output  PseudoPeriodic=off  Frequencies=[]  Unit=inherit  AffineConversion=off
      settings: SourceProductBaseCode=PW,SS
  Piston 1 Mass : fl_lib/Mechanical/Translational Elements/Mass  mass=tpc.mass1 kg  num_ports=foundation.enum.numPorts2.one  v_specify=off  v_priority=High  v=0 m/s  v_nominal_specify=off  v_nominal_unit=m/s  v_nominal_value=1  f_specify=off  f_priority=None  f=0 N  f_nominal_specify=off  f_nominal_unit=N  f_nominal_value=1
  Piston 2 Mass : fl_lib/Mechanical/Translational Elements/Mass  mass=tpc.mass2 kg  num_ports=foundation.enum.numPorts2.one  v_specify=off  v_priority=High  v=0 m/s  v_nominal_specify=off  v_nominal_unit=m/s  v_nominal_value=1  f_specify=off  f_priority=None  f=0 N  f_nominal_specify=off  f_nominal_unit=N  f_nominal_value=1
  R1/V1 : fl_lib/Isothermal Liquid/Elements/Reservoir (IL)  reservoir_type=foundation.enum.constant_controlled.constant  pressure_spec=foundation.enum.pressure_spec.atmospheric  reservoir_pressure=0.101325 MPa
      settings: SourceProductBaseCode=SS
  R2/V3 : fl_lib/Isothermal Liquid/Elements/Reservoir (IL)  reservoir_type=foundation.enum.constant_controlled.constant  pressure_spec=foundation.enum.pressure_spec.atmospheric  reservoir_pressure=0.101325 MPa
      settings: SourceProductBaseCode=SS
  Simulink-PS Converter : nesl_utility/Simulink-PS Converter  PhysicalDomain=network_engine_domain  SubClassName=ps_input  LeftPortType=input  RightPortType=output  PseudoPeriodic=off  Frequencies=[]  NoiseDistribution=none  NoiseParameters=[]  Unit=1  AffineConversion=off  FilteringAndDerivatives=filter  SimscapeFilterOrder=1  InputFilterTimeConstant=0.001  UdotUserProvided=0
      settings: SourceProductBaseCode=PW,SS
  Translational Hydro-Mechanical Converter1 : fl_lib/Isothermal Liquid/Elements/Translational Mechanical Converter (IL)  mech_orientation=foundation.enum.MechOrientationTranslational.Negative  displacement_spec=foundation.enum.DisplacementSpec.Calculate  x0=-(tpc.x13) m  interface_area=tpc.aPist m^2  dead_volume=tpc.v2D m^3  pressure_spec=foundation.enum.pressure_spec.atmospheric  environment_pressure=0.101325 MPa  dynamic_compressibility=simscape.enum.onoff.on  p0="tpc.pRes  Pa"
      settings: SourceProductBaseCode=SS  InternalSimscapePortConfiguration="{\"Bottom\":[],\"Left\":[{\"id\":\"A\",\"label\":\"A\",\"type\":\"foundation.isothermal_liquid.isothermal_liquid\"},{\"id\":\"C\",\"label\":\"C\",\"type\":\"foundation.mechanical.translational.translational\"}],\"Right\":[{\"id\":\"R\",\"label\":\"R\",\"type\":\"foundation.mechanical.translational.translational\"}],\"Top\":[]}"
  Translational Hydro-Mechanical Converter2 : fl_lib/Isothermal Liquid/Elements/Translational Mechanical Converter (IL)  mech_orientation=foundation.enum.MechOrientationTranslational.Negative  displacement_spec=foundation.enum.DisplacementSpec.Calculate  x0=-(tpc.x23) m  interface_area=tpc.aPist m^2  dead_volume=tpc.v4D m^3  pressure_spec=foundation.enum.pressure_spec.atmospheric  environment_pressure=0.101325 MPa  dynamic_compressibility=simscape.enum.onoff.on  p0=tpc.pRes Pa
      settings: SourceProductBaseCode=SS  InternalSimscapePortConfiguration="{\"Bottom\":[],\"Left\":[{\"id\":\"A\",\"label\":\"A\",\"type\":\"foundation.isothermal_liquid.isothermal_liquid\"},{\"id\":\"C\",\"label\":\"C\",\"type\":\"foundation.mechanical.translational.translational\"}],\"Right\":[{\"id\":\"R\",\"label\":\"R\",\"type\":\"foundation.mechanical.translational.translational\"}],\"Top\":[]}"
  Piston - Translational Motion 1 : PMIOPort  Side=Right
  Piston Translational Motion 2 : PMIOPort  Port=2  Side=Right
  Brake Circuit 1 : PMIOPort  Port=3  Side=Right
  Brake Circuit 2 : PMIOPort  Port=4  Side=Right
  FPR : Outport
  wires:
  Mux/1 -> Display/1
  PS-Simulink Converter/1 -> Mux/1
  PS-Simulink Converter1/1 -> Mux/2
  PS-Simulink Converter3/1 -> Mux1/2
  Mux1/1 -> Display1/1
  PS-Simulink Converter2/1 -> Mux1/1
  F/1 -> FPR/1, Simulink-PS Converter/1
  connections:
  R1/V1/LConn1 -- Compensating port 1/RConn1
  R2/V3/LConn1 -- Compensating port 2/RConn1
  Fixed Orifice1/RConn1 -- Brake Circuit 1/RConn1
  Fixed Orifice2/RConn1 -- Brake Circuit 2/RConn1
  K1/LConn1 -- Motion Sensor 1/LConn1 -- Translational Hydro-Mechanical Converter1/RConn1 -- Ideal Force Source/LConn1 -- Piston 1 Mass/LConn1 -- HD1/LConn1 -- C1/LConn1
  Fixed Orifice1/LConn1 -- Compensating port 1/LConn1 -- Translational Hydro-Mechanical Converter1/LConn1
  Piston 2 Mass/LConn1 -- Motion Sensor 2/LConn1 -- Translational Hydro-Mechanical Converter2/RConn1 -- C2/LConn1 -- K2/LConn1 -- HD2/LConn1 -- Translational Hydro-Mechanical Converter1/LConn2 -- C1/RConn1 -- K1/RConn1
  Translational Hydro-Mechanical Converter2/LConn1 -- Compensating port 2/LConn1 -- Fixed Orifice2/LConn1
  C2/RConn1 -- Motion Sensor 2/RConn2 -- Translational Hydro-Mechanical Converter2/LConn2 -- Ideal Force Source/RConn2 -- Motion Sensor 1/RConn1 -- Mechanical Translational Reference1/LConn1 -- HD1/RConn1 -- K2/RConn1 -- HD2/RConn1
  PS Lookup Table (1D)/LConn1 -- Piston Translational Motion 2/RConn1 -- PS-Simulink Converter2/LConn1 -- Motion Sensor 2/RConn1
  PS Lookup Table (1D)1/LConn1 -- PS-Simulink Converter/LConn1 -- Piston - Translational Motion 1/RConn1 -- Motion Sensor 1/RConn2
  PS Lookup Table (1D)1/RConn1 -- PS-Simulink Converter1/LConn1 -- Compensating port 1/LConn2
  PS Lookup Table (1D)/RConn1 -- PS-Simulink Converter3/LConn1 -- Compensating port 2/LConn2
  Simulink-PS Converter/RConn1 -- Ideal Force Source/RConn1

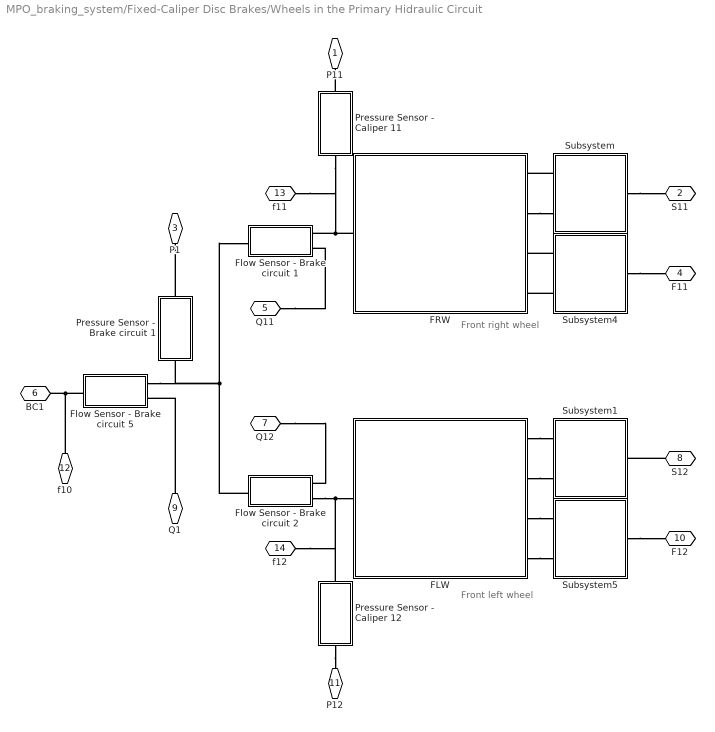
== system MPO_braking_system/Fixed-Caliper Disc Brakes/Wheels in the Primary Hidraulic Circuit ==
  note: Front right wheel
  note: Front left wheel
  FLW : Subsystem
      mask Display:
      | image('sdl_braking_caliper_disk_brake.png');
      | port_label('LConn',1,'Brk1')
      | port_label('RConn',1,'CPTM1')
      | port_label('RConn',2,'CPTM2')
      | port_label('RConn',3,'CPF1')
      | port_label('RConn',4,'CPF2')
  FRW : Subsystem
      mask Display:
      | image('sdl_braking_caliper_disk_brake.png');
      | port_label('LConn',1,'Brk1')
      | port_label('RConn',1,'CPTM1')
      | port_label('RConn',2,'CPTM2')
      | port_label('RConn',3,'CPF1')
      | port_label('RConn',4,'CPF2')
  Flow Sensor - Brake circuit 1 : Subsystem
  Flow Sensor - Brake circuit 2 : Subsystem
  Flow Sensor - Brake circuit 5 : Subsystem
  Pressure Sensor - Brake circuit 1 : Subsystem
  Pressure Sensor - Caliper 11 : Subsystem
  Pressure Sensor - Caliper 12 : Subsystem
  Subsystem : Subsystem
  Subsystem1 : Subsystem
  Subsystem4 : Subsystem
  Subsystem5 : Subsystem
  P11 : PMIOPort  Side=Right
  S11 : PMIOPort  Port=2  Side=Right
  P1 : PMIOPort  Port=3  Side=Right
  F11 : PMIOPort  Port=4  Side=Right
  Q11 : PMIOPort  Port=5  Side=Right
  BC1 : PMIOPort  Port=6  Side=Left
  Q12 : PMIOPort  Port=7  Side=Right
  S12 : PMIOPort  Port=8  Side=Right
  Q1 : PMIOPort  Port=9  Side=Right
  F12 : PMIOPort  Port=10  Side=Right
  P12 : PMIOPort  Port=11  Side=Right
  f10 : PMIOPort  Port=12  Side=Left
  f11 : PMIOPort  Port=13  Side=Left
  f12 : PMIOPort  Port=14  Side=Left
  connections:
  Pressure Sensor - Brake circuit 1/RConn1 -- P1/RConn1
  Subsystem/RConn1 -- S11/RConn1
  Subsystem4/RConn1 -- F11/RConn1
  Subsystem5/RConn1 -- F12/RConn1
  FLW/RConn3 -- Subsystem5/LConn1
  Subsystem/LConn1 -- FRW/RConn1
  FLW/RConn1 -- Subsystem1/LConn1
  Flow Sensor - Brake circuit 2/LConn1 -- Flow Sensor - Brake circuit 5/RConn1 -- Pressure Sensor - Brake circuit 1/LConn1 -- Flow Sensor - Brake circuit 1/LConn1
  Subsystem4/LConn1 -- FRW/RConn3
  Flow Sensor - Brake circuit 2/RConn2 -- f12/RConn1 -- Pressure Sensor - Caliper 12/LConn1 -- FLW/LConn1
  FLW/RConn4 -- Subsystem5/LConn2
  Q12/RConn1 -- Flow Sensor - Brake circuit 2/RConn1
  Subsystem4/LConn2 -- FRW/RConn4
  FLW/RConn2 -- Subsystem1/LConn2
  S12/RConn1 -- Subsystem1/RConn1
  Flow Sensor - Brake circuit 5/LConn1 -- f10/RConn1 -- BC1/RConn1
  Pressure Sensor - Caliper 11/RConn1 -- P11/RConn1
  FRW/LConn1 -- Pressure Sensor - Caliper 11/LConn1 -- f11/RConn1 -- Flow Sensor - Brake circuit 1/RConn1
  Q1/RConn1 -- Flow Sensor - Brake circuit 5/RConn2
  FRW/RConn2 -- Subsystem/LConn2
  Pressure Sensor - Caliper 12/RConn1 -- P12/RConn1
  Q11/RConn1 -- Flow Sensor - Brake circuit 1/RConn2

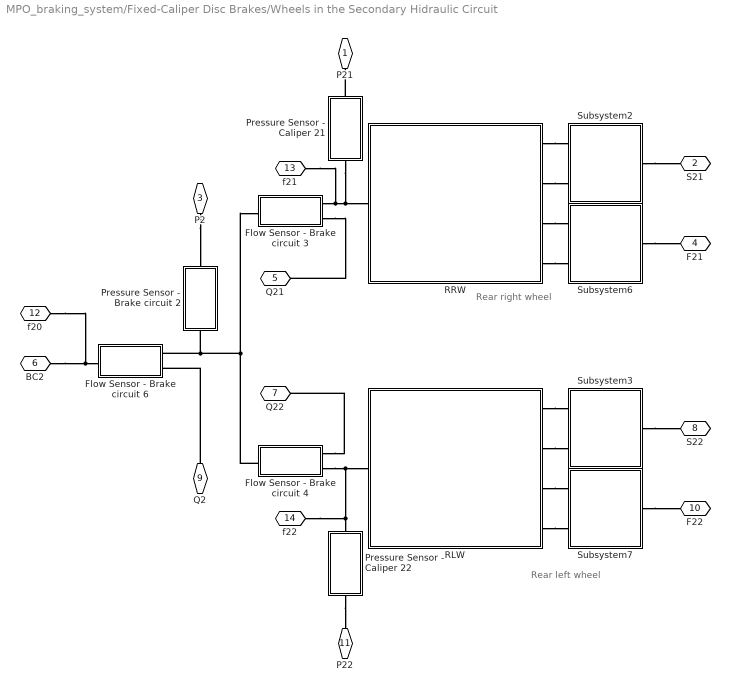
== system MPO_braking_system/Fixed-Caliper Disc Brakes/Wheels in the Secondary Hidraulic Circuit ==
  note: Rear right wheel
  note: Rear left wheel
  Flow Sensor - Brake circuit 3 : Subsystem
  Flow Sensor - Brake circuit 4 : Subsystem
  Flow Sensor - Brake circuit 6 : Subsystem
  Pressure Sensor - Brake circuit 2 : Subsystem
  Pressure Sensor - Caliper 21 : Subsystem
  Pressure Sensor - Caliper 22 : Subsystem
  RLW : Subsystem
      mask Display:
      | image('sdl_braking_caliper_disk_brake.png');
      | port_label('LConn',1,'Brk1')
      | port_label('RConn',1,'CPTM1')
      | port_label('RConn',2,'CPTM2')
      | port_label('RConn',3,'CPF1')
      | port_label('RConn',4,'CPF2')
  RRW : Subsystem
      mask Display:
      | image('sdl_braking_caliper_disk_brake.png');
      | port_label('LConn',1,'Brk1')
      | port_label('RConn',1,'CPTM1')
      | port_label('RConn',2,'CPTM2')
      | port_label('RConn',3,'CPF1')
      | port_label('RConn',4,'CPF2')
  Subsystem2 : Subsystem
  Subsystem3 : Subsystem
  Subsystem6 : Subsystem
  Subsystem7 : Subsystem
  P21 : PMIOPort  Side=Right
  S21 : PMIOPort  Port=2  Side=Right
  P2 : PMIOPort  Port=3  Side=Right
  F21 : PMIOPort  Port=4  Side=Right
  Q21 : PMIOPort  Port=5  Side=Right
  BC2 : PMIOPort  Port=6  Side=Left
  Q22 : PMIOPort  Port=7  Side=Right
  S22 : PMIOPort  Port=8  Side=Right
  Q2 : PMIOPort  Port=9  Side=Right
  F22 : PMIOPort  Port=10  Side=Right
  P22 : PMIOPort  Port=11  Side=Right
  f20 : PMIOPort  Port=12  Side=Left
  f21 : PMIOPort  Port=13  Side=Left
  f22 : PMIOPort  Port=14  Side=Left
  connections:
  RRW/RConn1 -- Subsystem2/LConn1
  RRW/RConn2 -- Subsystem2/LConn2
  Subsystem2/RConn1 -- S21/RConn1
  RLW/RConn2 -- Subsystem3/LConn2
  Flow Sensor - Brake circuit 6/LConn1 -- f20/RConn1 -- BC2/RConn1
  RLW/RConn1 -- Subsystem3/LConn1
  Subsystem3/RConn1 -- S22/RConn1
  RRW/RConn4 -- Subsystem6/LConn2
  Subsystem7/RConn1 -- F22/RConn1
  Flow Sensor - Brake circuit 4/RConn2 -- f22/RConn1 -- Pressure Sensor - Caliper 22/LConn1 -- RLW/LConn1
  RLW/RConn4 -- Subsystem7/LConn2
  RLW/RConn3 -- Subsystem7/LConn1
  Subsystem6/RConn1 -- F21/RConn1
  Flow Sensor - Brake circuit 4/RConn1 -- Q22/RConn1
  Flow Sensor - Brake circuit 3/RConn1 -- f21/RConn1 -- Pressure Sensor - Caliper 21/LConn1 -- RRW/LConn1
  Pressure Sensor - Brake circuit 2/LConn1 -- Flow Sensor - Brake circuit 6/RConn1 -- Flow Sensor - Brake circuit 4/LConn1 -- Flow Sensor - Brake circuit 3/LConn1
  RRW/RConn3 -- Subsystem6/LConn1
  Flow Sensor - Brake circuit 3/RConn2 -- Q21/RConn1
  P2/RConn1 -- Pressure Sensor - Brake circuit 2/RConn1
  Pressure Sensor - Caliper 22/RConn1 -- P22/RConn1
  Q2/RConn1 -- Flow Sensor - Brake circuit 6/RConn2
  Pressure Sensor - Caliper 21/RConn1 -- P21/RConn1

== system MPO_braking_system/Tandem Master Cylinder/Motion Sensor 1 ==
  Ideal Translational Motion Sensor : fl_lib/Mechanical/Mechanical Sensors/Ideal Translational Motion Sensor  offset=0 m
  PS Terminator1 : fl_lib/Physical Signals/Sinks/PS Terminator
  C : PMIOPort  Side=Right
  P : PMIOPort  Port=2  Side=Right
  R : PMIOPort  Port=3  Side=Left
  connections:
  PS Terminator1/LConn1 -- Ideal Translational Motion Sensor/RConn2
  Ideal Translational Motion Sensor/LConn1 -- R/RConn1
  Ideal Translational Motion Sensor/RConn3 -- P/RConn1
  Ideal Translational Motion Sensor/RConn1 -- C/RConn1

== system MPO_braking_system/Tandem Master Cylinder/Motion Sensor 2 ==
  Ideal Translational Motion Sensor : fl_lib/Mechanical/Mechanical Sensors/Ideal Translational Motion Sensor  offset=0 m
  PS Terminator : fl_lib/Physical Signals/Sinks/PS Terminator
  P : PMIOPort  Side=Right
  C : PMIOPort  Port=2  Side=Right
  R : PMIOPort  Port=3  Side=Left
  connections:
  PS Terminator/LConn1 -- Ideal Translational Motion Sensor/RConn2
  Ideal Translational Motion Sensor/RConn3 -- P/RConn1
  Ideal Translational Motion Sensor/RConn1 -- C/RConn1
  Ideal Translational Motion Sensor/LConn1 -- R/RConn1
